simulink model "task_A1_mod"  (R2013b)
settings: Solver=ode45  StartTime=0.0  StopTime=10.0  RelTol=1e-3
values from neighbouring files (symbols this model uses):
  a0 = 8*lamda/(c*ro*(b-a)^2)    [task_A_scr.m]    (also in task_B_scr.m = 8*lamda/(3*c*ro*(b-a)^2); task_C_scr.m = 4*lamda*(2-A1-B1)/(c*ro*(b-a)^2))
  b0 = a0/2    [task_A_scr.m]    (also in task_B_scr.m)
  T_a = 350    [task_A_scr.m]    (also in task_C_scr.m = 600)
  T_b = 400    [task_A_scr.m]    (also in task_B_scr.m = 350; task_C_scr.m = 300)
undefined symbols (not defined in the file or in its folder): T_0
settings Model: Creator=Yurii  LastModifiedBy=Yurii

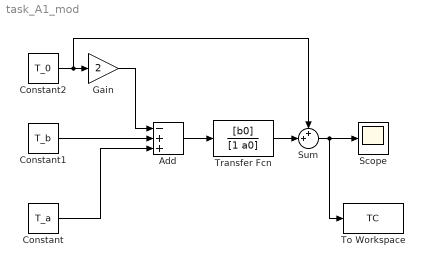
== system task_A1_mod ==
  Add : Sum  Inputs=-++
  Constant : Constant  Value=T_a
  Constant1 : Constant  Value=T_b
  Constant2 : Constant  Value=T_0
  Gain : Gain  Gain=2
  Scope : Scope
  Sum : Sum  Inputs=++|
  To Workspace : ToWorkspace  VariableName=TC  SampleTime=-1  SaveFormat=Timeseries
  Transfer Fcn : TransferFcn  Numerator=[b0]  Denominator=[1 a0]
  wires:
  Constant/1 -> Add/3
  Constant1/1 -> Add/2
  Constant2/1 -> Sum/1, Gain/1
  Gain/1 -> Add/1
  Add/1 -> Transfer Fcn/1
  Transfer Fcn/1 -> Sum/2
  Sum/1 -> To Workspace/1, Scope/1
